simulink model "Data_generation_simulink"  (R2021a)
settings: Solver=VariableStepAuto  StartTime=0.0  StopTime=(s-1)*h  RelTol=1e-3
InitFcn:
  | clss1
values from neighbouring files (symbols this model uses):
  C_c = -C_c    [clss1.m]
  D_c = -D_c    [clss1.m]
  h = 0.02    [clss1.m]
undefined symbols (not defined in the file or in its folder): A_c, B_c
settings Model: Creator=Maik1  LastModifiedBy=chidi
settings SolverCC: AlgebraicLoopSolver=TrustRegion
settings DataIOCC: ReturnWorkspaceOutputs=off
settings DebuggingCC: SFMachineParentedDataDiag=warning  ArithmeticOperatorsInVariantConditions=warning
settings SFSimCC: CustomCodeUndefinedFunction=UseInterfaceOnly

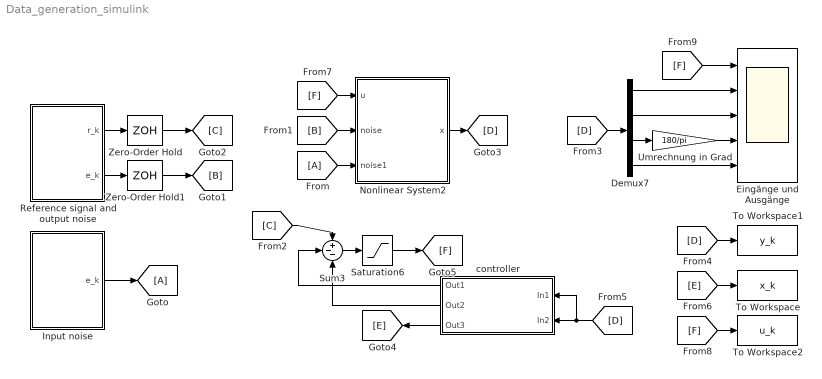
== system Data_generation_simulink ==
  Demux7 : Demux
  Eingänge und Ausgänge : Scope  NumInputPorts=5
  Input noise : MATLAB Function  TreatAsAtomicUnit=on
  Nonlinear System2 : Subsystem
  Reference signal and output noise : MATLAB Function  TreatAsAtomicUnit=on
  Saturation6 : Saturate  UpperLimit=10  LowerLimit=-10
  Sum3 : Sum  Inputs=+--
  To Workspace : ToWorkspace  VariableName=x_k  SampleTime=-1
  To Workspace1 : ToWorkspace  VariableName=y_k  SampleTime=-1
      settings: Save2DSignal=2-D array (concatenate along first dimension)
  To Workspace2 : ToWorkspace  VariableName=u_k  SampleTime=-1
      settings: Save2DSignal=2-D array (concatenate along first dimension)
  Umrechnung in Grad : Gain  Gain=180/pi
  Zero-Order Hold : ZeroOrderHold  SampleTime=h
  Zero-Order Hold1 : ZeroOrderHold  SampleTime=h
  controller : Subsystem
  wires:
  Reference signal and output noise/1(r_k) -> Zero-Order Hold/1
  Reference signal and output noise/2(e_k) -> Zero-Order Hold1/1
  Demux7/3 -> Umrechnung in Grad/1
  Sum3/1 -> Saturation6/1
  Demux7/4 -> Eingänge und Ausgänge/5
  Demux7/1 -> Eingänge und Ausgänge/2
  Demux7/2 -> Eingänge und Ausgänge/3
  Umrechnung in Grad/1 -> Eingänge und Ausgänge/4
  Input noise/1(e_k) -> [A]
  [A] -> Nonlinear System2/3(noise1)
  Zero-Order Hold1/1 -> [B]
  [B] -> Nonlinear System2/2(noise)
  Zero-Order Hold/1 -> [C]
  [C] -> Sum3/1
  controller/1(Out1) -> Sum3/2
  controller/2(Out2) -> Sum3/3
  controller/3(Out3) -> [E]
  Nonlinear System2/1(x) -> [D]
  [D] -> Demux7/1
  [D] -> To Workspace1/1
  [D] -> controller/1(In1), controller/2(In2)
  [E] -> To Workspace/1
  Saturation6/1 -> [F]
  [F] -> Nonlinear System2/1(u)
  [F] -> To Workspace2/1
  [F] -> Eingänge und Ausgänge/1

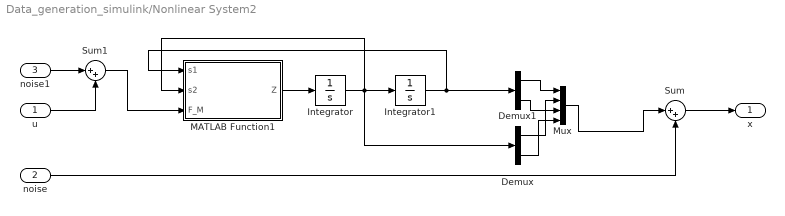
== system Data_generation_simulink/Nonlinear System2 ==
  u : Inport
  noise : Inport  Port=2
  noise1 : Inport  Port=3
  Demux : Demux  Outputs=2
  Demux1 : Demux  Outputs=2
  Integrator : Integrator  InitialCondition=[0; 0]
  Integrator1 : Integrator  InitialCondition=[0;0.1 ]
  MATLAB Function1 : MATLAB Function  TreatAsAtomicUnit=on
  Mux : Mux
  Sum : Sum  Inputs=|++
  Sum1 : Sum  Inputs=|++
  x : Outport
  wires:
  Integrator1/1 -> Demux1/1, MATLAB Function1/1(s1)
  MATLAB Function1/1(Z) -> Integrator/1
  Integrator/1 -> Demux/1, Integrator1/1, MATLAB Function1/2(s2)
  u/1 -> Sum1/2
  Demux1/1 -> Mux/1
  Demux1/2 -> Mux/3
  Demux/1 -> Mux/2
  Demux/2 -> Mux/4
  Mux/1 -> Sum/1
  Sum/1 -> x/1
  noise/1 -> Sum/2
  Sum1/1 -> MATLAB Function1/3(F_M)
  noise1/1 -> Sum1/1

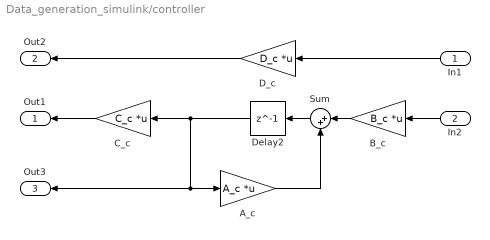
== system Data_generation_simulink/controller ==
  In1 : Inport
  In2 : Inport  Port=2
  A_c : Gain  Gain=A_c  Multiplication=Matrix(K*u)
  B_c : Gain  Gain=B_c  Multiplication=Matrix(K*u)
  C_c : Gain  Gain=C_c  Multiplication=Matrix(K*u)
  D_c : Gain  Gain=D_c  Multiplication=Matrix(K*u)
  Delay2 : Delay  DelayLength=1  InitialCondition=0
  Sum : Sum  Inputs=|++
  Out1 : Outport
  Out2 : Outport  Port=2
  Out3 : Outport  Port=3
  wires:
  In2/1 -> B_c/1
  B_c/1 -> Sum/1
  D_c/1 -> Out2/1
  A_c/1 -> Sum/2
  C_c/1 -> Out1/1
  Sum/1 -> Delay2/1
  Delay2/1 -> A_c/1, Out3/1, C_c/1
  In1/1 -> D_c/1

== matlab function Data_generation_simulink/Input noise ==
  data: e_k output
function e_k  = fcn
e_k = 1/10*randn(1,1);
e_k(1) = e_k(1)/10;

== matlab function Data_generation_simulink/Reference signal and output noise ==
  data: r_k output; e_k output
function [r_k,e_k] = fcn
r_k = 1*randn(1,1);
e_k = 1/10*randn(4,1);
e_k(1) = e_k(1)/10;
e_k(2) = e_k(2)/10;
e_k(3) = e_k(3)/180*pi;
e_k(4) = e_k(4)/180*pi;

== matlab function Data_generation_simulink/Nonlinear System2/MATLAB Function1 ==
  data: s1 input; s2 input; Z output; F_M input
%% System dynamic des Pendels
function Z = pendel(s1,s2,F_M)
%T_sample = 0.01;
x = s1(1);
x_d = s2(1);
phi = s1(2);
phi_d = s2(2);


% Systemparameters
m_p = 0.329;
m_w = 3.2;
l_sp = 0.488;
f_w = 6.2;
f_p = 0.009;
g = 9.81;
J_A = 0.0743;

% Dynamic des Wagens
x_dd = (m_w + m_p) \ F_M - f_w / (m_w + m_p) * x_d;

% x_d = x_d + x_dd * T_sample;
% x = x + x_d *T_sample;

% Dynamic des Pendels
phi_dd = -(m_p * l_sp) / J_A * x_dd * cos(phi) + m_p * g * l_sp / J_A * sin(phi) - f_p / J_A * phi_d;
% phi_d = phi_d + phi_dd * T_sample;
% phi = phi + phi_d * T_sample; 


if abs(phi) > pi
    phi = -sign(phi)*(2*pi-abs(phi));
end


Z = [x_dd;phi_dd];

end
